simulink model "gyro_data_test"  (R2019a)
settings: Solver=FixedStepAuto  StartTime=0.0  StopTime=10  FixedStep=0.001  RelTol=1e-3
settings Model: Creator=asmialek  LastModifiedBy=asmialek

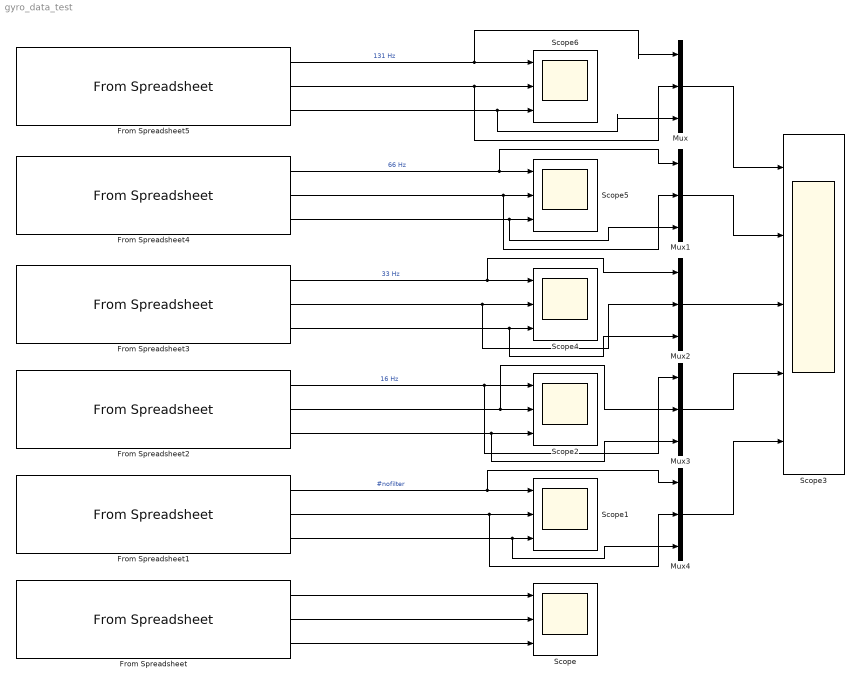
== system gyro_data_test ==
  From Spreadsheet : FromSpreadsheet  FileName=/home/asmialek/Projects/BEXUS/irisc-control/gyro_data/gyro_data2_new_new.xlsx
  From Spreadsheet1 : FromSpreadsheet  FileName=/home/asmialek/Projects/BEXUS/irisc-control/gyro_data/gyro_data2_new.xlsx
  From Spreadsheet2 : FromSpreadsheet  FileName=/home/asmialek/Projects/BEXUS/irisc-control/gyro_data/gyro_16HzLP_new.xlsx
  From Spreadsheet3 : FromSpreadsheet  FileName=/home/asmialek/Projects/BEXUS/irisc-control/gyro_data/gyro_33HzLP_new.xlsx
  From Spreadsheet4 : FromSpreadsheet  FileName=/home/asmialek/Projects/BEXUS/irisc-control/gyro_data/gyro_66HzLP_new.xlsx
  From Spreadsheet5 : FromSpreadsheet  FileName=/home/asmialek/Projects/BEXUS/irisc-control/gyro_data/gyro_131HzLP_new.xlsx
  Mux{,1..4} (5 alike) : Mux  Inputs=3
  Scope{,1..2,4..6} (6 alike) : Scope  NumInputPorts=3
  Scope3 : Scope  NumInputPorts=5
  wires:
  From Spreadsheet/1 -> Scope/1
  From Spreadsheet/2 -> Scope/2
  From Spreadsheet/3 -> Scope/3
  From Spreadsheet1/1 -> Mux4/1, Scope1/1  "#nofilter"
  From Spreadsheet1/2 -> Mux4/2, Scope1/2
  From Spreadsheet1/3 -> Mux4/3, Scope1/3
  From Spreadsheet2/1 -> Mux3/1, Scope2/1  "16 Hz"
  From Spreadsheet2/2 -> Mux3/2, Scope2/2
  From Spreadsheet2/3 -> Mux3/3, Scope2/3
  From Spreadsheet3/3 -> Mux2/3, Scope4/3
  From Spreadsheet3/1 -> Mux2/1, Scope4/1  "33 Hz"
  From Spreadsheet3/2 -> Mux2/2, Scope4/2
  From Spreadsheet4/3 -> Mux1/3, Scope5/3
  From Spreadsheet4/1 -> Mux1/1, Scope5/1  "66 Hz"
  From Spreadsheet4/2 -> Mux1/2, Scope5/2
  From Spreadsheet5/3 -> Mux/3, Scope6/3
  From Spreadsheet5/2 -> Mux/2, Scope6/2
  From Spreadsheet5/1 -> Mux/1, Scope6/1  "131 Hz"
  Mux/1 -> Scope3/1
  Mux1/1 -> Scope3/2
  Mux2/1 -> Scope3/3
  Mux3/1 -> Scope3/4
  Mux4/1 -> Scope3/5
